simulink model "bms_master"  (R2024b)
settings: Solver=FixedStepDiscrete  StartTime=0.0  StopTime=T_stop  FixedStep=0.1  RelTol=1e-3
undefined symbols (not defined in the file): bms, C1_data, C2_data, dt, ekf_params, OCV_data, P_chiller_max, P_heater_max, Q_nom_Ah, R0_data, R1_data, R2_data, SoC_bp_ecm, SoC_bp_ocv, T_bp, T_cool_off, T_cool_on, T_cool_target, T_heat_off, T_heat_on, T_heat_target
libraries: simulink x28, components x12
settings Model: DataDictionary=buses.sldd  Creator=rayen  LastModifiedBy=rayen
settings OptimizationCC: DefaultParameterBehavior=Inlined  EnhancedBackFolding=on  PassReuseOutputArgsAs=Individual arguments  ZeroExternalMemoryAtStartup=off  ZeroInternalMemoryAtStartup=off  OptimizeBlockOrder=speed  DifferentSizesBufferReuse=on  OptimizationCustomize=off  EfficientTunableParamExpr=on
settings DebuggingCC: AlgebraicLoopMsg=error  ParameterTunabilityLossMsg=error
settings HardwareCC: TargetBitPerPointer=64  TargetBitPerSizeT=64  TargetBitPerPtrDiffT=64  TargetLargestAtomicFloat=Float  TargetIntDivRoundTo=Zero  TargetEndianess=LittleEndian  TargetWordSize=64  TargetHWDeviceType=Intel->x86-64 (Windows64)  ProdEqTarget=off
settings SFSimCC: MATLABDynamicMemAlloc=off  SimTargetLang=C++
settings RTWCC: Description=Embedded Coder  SystemTargetFile=ert.tlc  TemplateMakefile=ert_default_tmf
settings CodeAppCC: ForceParamTrailComments=on  IgnoreCustomStorageClasses=off  OperatorAnnotations=on  SimulinkDataObjDesc=on  SFDataObjDesc=on  InsertBlockDesc=on
settings ERTTargetCC: TargetLangStandard=C99 (ISO)  GenerateSampleERTMain=on  ERTCustomFileTemplate=example_file_process.tlc

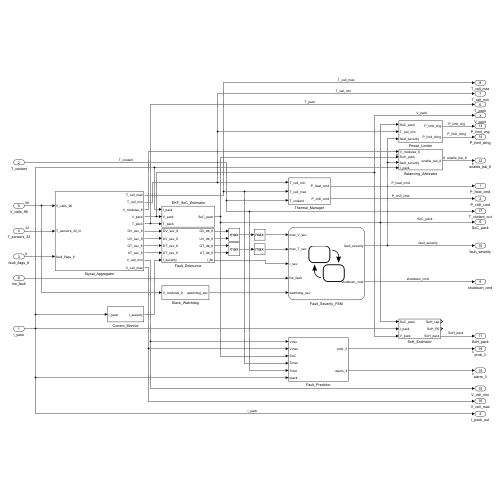
[thumbnail: Simulink's stored preview of the top-level diagram]
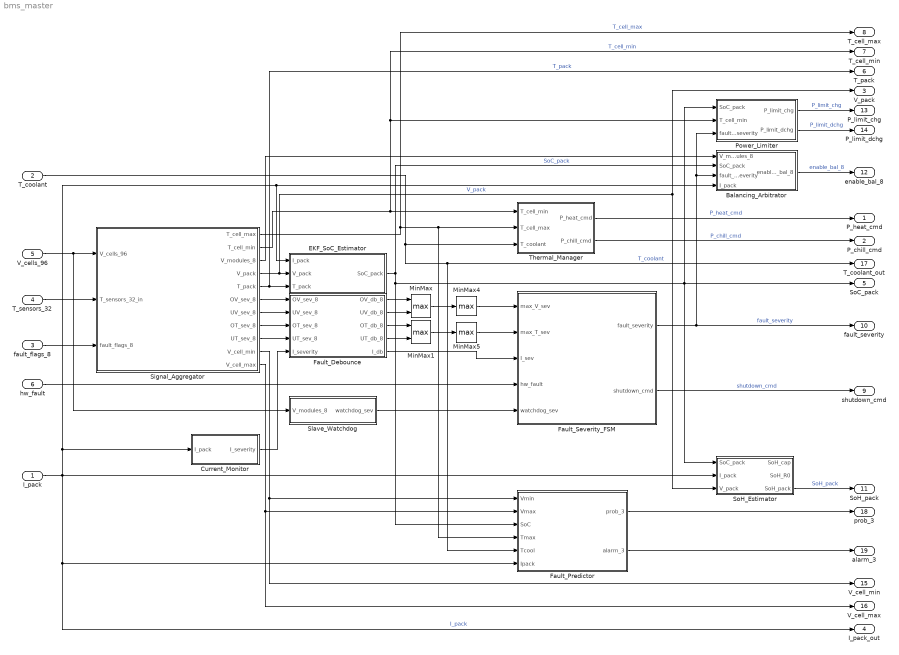
== system bms_master ==
  I_pack : Inport  OutDataTypeStr=double  PortDimensions=1
  T_coolant : Inport  Port=2  OutDataTypeStr=double  PortDimensions=1
  fault_flags_8 : Inport  Port=3  OutDataTypeStr=double  PortDimensions=[8]
  T_sensors_32 : Inport  Port=4  OutDataTypeStr=double  PortDimensions=[32]
  V_cells_96 : Inport  Port=5  OutDataTypeStr=double  PortDimensions=[96]
  hw_fault : Inport  Port=6
  " EKF_SoC_Estimator" : Subsystem
  Balancing_Arbitrator : Subsystem
  Current_Monitor : Subsystem
  Fault_Debounce : Subsystem
  Fault_Predictor : Subsystem
  Fault_Severity_FSM : Stateflow chart  TreatAsAtomicUnit=on
  MinMax : MinMax  Function=max  Inputs=2
  MinMax1 : MinMax  Function=max  Inputs=2
  MinMax4 : MinMax  Function=max
  MinMax5 : MinMax  Function=max
  Power_Limiter : Subsystem
  Signal_Aggregator : Subsystem
  Slave_Watchdog : Subsystem
  SoH_Estimator : Subsystem
  Thermal_Manager : Subsystem
  P_heat_cmd : Outport  OutDataTypeStr=double  PortDimensions=1
  P_chill_cmd : Outport  Port=2  OutDataTypeStr=double  PortDimensions=1
  V_pack : Outport  Port=3  OutDataTypeStr=double  PortDimensions=1
  I_pack_out : Outport  Port=4  OutDataTypeStr=double  PortDimensions=1
  SoC_pack : Outport  Port=5  OutDataTypeStr=double  PortDimensions=1
  T_pack : Outport  Port=6  OutDataTypeStr=double  PortDimensions=1
  T_cell_min : Outport  Port=7  OutDataTypeStr=double  PortDimensions=1
  T_cell_max : Outport  Port=8  OutDataTypeStr=double  PortDimensions=1
  shutdown_cmd : Outport  Port=9  OutDataTypeStr=double  PortDimensions=1
  fault_severity : Outport  Port=10  OutDataTypeStr=double  PortDimensions=1
  SoH_pack : Outport  Port=11  OutDataTypeStr=double  PortDimensions=1
  enable_bal_8 : Outport  Port=12  OutDataTypeStr=double  PortDimensions=[8]
  P_limit_chg : Outport  Port=13  OutDataTypeStr=double  PortDimensions=1
  P_limit_dchg : Outport  Port=14  OutDataTypeStr=double  PortDimensions=1
  V_cell_min : Outport  Port=15
  V_cell_max : Outport  Port=16
  T_coolant_out : Outport  Port=17
  prob_3 : Outport  Port=18  PortDimensions=[3]
  alarm_3 : Outport  Port=19  PortDimensions=[3]
  wires:
  Signal_Aggregator/6(OV_sev_8) -> Fault_Debounce/1(OV_sev_8)
  Signal_Aggregator/7(UV_sev_8) -> Fault_Debounce/2(UV_sev_8)
  Signal_Aggregator/8(OT_sev_8) -> Fault_Debounce/3(OT_sev_8)
  Signal_Aggregator/9(UT_sev_8) -> Fault_Debounce/4(UT_sev_8)
  Fault_Debounce/1(OV_db_8) -> MinMax/1
  Fault_Debounce/2(UV_db_8) -> MinMax/2
  Fault_Debounce/3(OT_db_8) -> MinMax1/1
  Fault_Debounce/4(UT_db_8) -> MinMax1/2
  MinMax/1 -> MinMax4/1
  MinMax1/1 -> MinMax5/1
  MinMax4/1 -> Fault_Severity_FSM/1(max_V_sev)
  MinMax5/1 -> Fault_Severity_FSM/2(max_T_sev)
  Slave_Watchdog/1(watchdog_sev) -> Fault_Severity_FSM/5(watchdog_sev)
  Signal_Aggregator/2(T_cell_min) -> Thermal_Manager/1(T_cell_min), T_cell_min/1, Power_Limiter/2(T_cell_min)  "T_cell_min"
  Signal_Aggregator/1(T_cell_max) -> T_cell_max/1, Thermal_Manager/2(T_cell_max), Fault_Predictor/4(Tmax)  "T_cell_max"
  Thermal_Manager/1(P_heat_cmd) -> P_heat_cmd/1  "P_heat_cmd"
  Thermal_Manager/2(P_chill_cmd) -> P_chill_cmd/1  "P_chill_cmd"
  T_coolant/1 -> Fault_Predictor/5(Tcool), T_coolant_out/1, Thermal_Manager/3(T_coolant)  "T_coolant"
  Signal_Aggregator/3(V_modules_8) -> Balancing_Arbitrator/1(V_modules_8)
  Fault_Severity_FSM/1(fault_severity) -> fault_severity/1, Power_Limiter/3(fault_severity), Balancing_Arbitrator/3(fault_severity)  "fault_severity"
  I_pack/1 -> I_pack_out/1, Fault_Predictor/6(Ipack), Current_Monitor/1(I_pack), Balancing_Arbitrator/4(I_pack), " EKF_SoC_Estimator"/1(I_pack), SoH_Estimator/2(I_pack)  "I_pack"
  Balancing_Arbitrator/1(enable_bal_8) -> enable_bal_8/1  "enable_bal_8"
  " EKF_SoC_Estimator"/1(SoC_pack) -> Fault_Predictor/3(SoC), Power_Limiter/1(SoC_pack), SoH_Estimator/1(SoC_pack), SoC_pack/1, Balancing_Arbitrator/2(SoC_pack)  "SoC_pack"
  Power_Limiter/1(P_limit_chg) -> P_limit_chg/1  "P_limit_chg"
  Power_Limiter/2(P_limit_dchg) -> P_limit_dchg/1  "P_limit_dchg"
  Fault_Severity_FSM/2(shutdown_cmd) -> shutdown_cmd/1  "shutdown_cmd"
  Signal_Aggregator/4(V_pack) -> " EKF_SoC_Estimator"/2(V_pack), SoH_Estimator/3(V_pack), V_pack/1  "V_pack"
  SoH_Estimator/3(SoH_pack) -> SoH_pack/1  "SoH_pack"
  Signal_Aggregator/5(T_pack) -> T_pack/1, " EKF_SoC_Estimator"/3(T_pack)  "T_pack"
  V_cells_96/1 -> Slave_Watchdog/1(V_modules_8), Signal_Aggregator/1(V_cells_96)
  Fault_Debounce/5(I_db) -> Fault_Severity_FSM/3(I_sev)
  T_sensors_32/1 -> Signal_Aggregator/2(T_sensors_32_in)
  fault_flags_8/1 -> Signal_Aggregator/3(fault_flags_8)
  hw_fault/1 -> Fault_Severity_FSM/4(hw_fault)
  Signal_Aggregator/11(V_cell_max) -> Fault_Predictor/2(Vmax), V_cell_max/1
  Signal_Aggregator/10(V_cell_min) -> Fault_Predictor/1(Vmin), V_cell_min/1
  Current_Monitor/1(I_severity) -> Fault_Debounce/5(I_severity)
  Fault_Predictor/1(prob_3) -> prob_3/1
  Fault_Predictor/2(alarm_3) -> alarm_3/1

== system bms_master/ EKF_SoC_Estimator ==
  I_pack : Inport
  V_pack : Inport  Port=2
  T_pack : Inport  Port=3
  Constant : Constant  Value=96
  MATLAB Function : MATLAB Function  TreatAsAtomicUnit=on
  SoC_pack : Outport
  wires:
  V_pack/1 -> MATLAB Function/1(V_pack)
  I_pack/1 -> MATLAB Function/2(I_pack)
  T_pack/1 -> MATLAB Function/3(T_pack)
  MATLAB Function/1(SoC_pack) -> SoC_pack/1
  Constant/1 -> MATLAB Function/4(N_series)

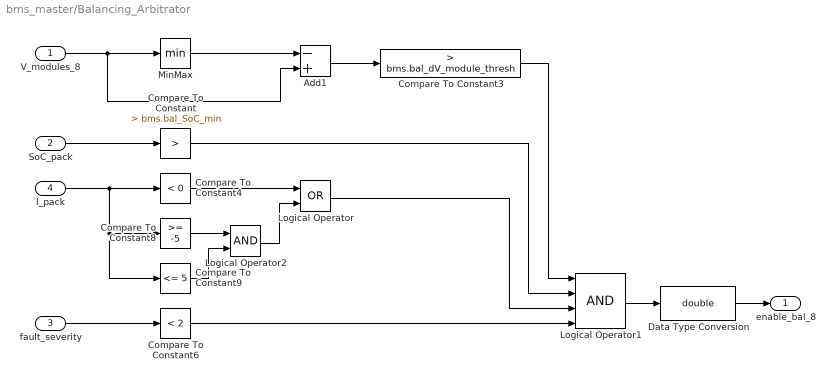
== system bms_master/Balancing_Arbitrator ==
  V_modules_8 : Inport  PortDimensions=[8]
  SoC_pack : Inport  Port=2
  fault_severity : Inport  Port=3  PortDimensions=[1]
  I_pack : Inport  Port=4
  Add1 : Sum  Inputs=-+
  Compare To Constant : simulink/Logic and Bit Operations/Compare To Constant  relop=>  const=bms.bal_SoC_min  OutDataTypeStr=boolean
  Compare To Constant3 : simulink/Logic and Bit Operations/Compare To Constant  relop=>  const=bms.bal_dV_module_thresh  OutDataTypeStr=boolean
  Compare To Constant4 : simulink/Logic and Bit Operations/Compare To Constant  relop=<  const=0  OutDataTypeStr=boolean
  Compare To Constant6 : simulink/Logic and Bit Operations/Compare To Constant  relop=<  const=2  OutDataTypeStr=boolean
  Compare To Constant8 : simulink/Logic and Bit Operations/Compare To Constant  relop=>=  const=-5  OutDataTypeStr=boolean
  Compare To Constant9 : simulink/Logic and Bit Operations/Compare To Constant  relop=<=  const=5  OutDataTypeStr=boolean
  Data Type Conversion : DataTypeConversion  OutDataTypeStr=double  SaturateOnIntegerOverflow=off  RndMeth=Floor
  Logical Operator : Logic  Operator=OR  AllPortsSameDT=off  OutDataTypeStr=boolean
  Logical Operator1 : Logic  Inputs=4  AllPortsSameDT=off  OutDataTypeStr=boolean
  Logical Operator2 : Logic  AllPortsSameDT=off  OutDataTypeStr=boolean
  MinMax : MinMax
  enable_bal_8 : Outport  PortDimensions=[8]
  wires:
  SoC_pack/1 -> Compare To Constant/1
  V_modules_8/1 -> MinMax/1, Add1/2
  I_pack/1 -> Compare To Constant9/1, Compare To Constant8/1, Compare To Constant4/1
  fault_severity/1 -> Compare To Constant6/1
  Compare To Constant8/1 -> Logical Operator2/1
  Compare To Constant9/1 -> Logical Operator2/2
  Compare To Constant4/1 -> Logical Operator/1
  Logical Operator2/1 -> Logical Operator/2
  Logical Operator1/1 -> Data Type Conversion/1
  Data Type Conversion/1 -> enable_bal_8/1
  MinMax/1 -> Add1/1
  Add1/1 -> Compare To Constant3/1
  Compare To Constant6/1 -> Logical Operator1/4
  Compare To Constant3/1 -> Logical Operator1/1
  Compare To Constant/1 -> Logical Operator1/2
  Logical Operator/1 -> Logical Operator1/3

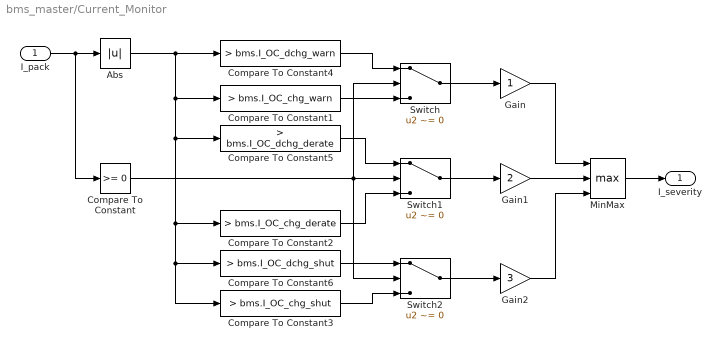
== system bms_master/Current_Monitor ==
  I_pack : Inport
  Abs : Abs  SaturateOnIntegerOverflow=off
  Compare To Constant : simulink/Logic and Bit Operations/Compare To Constant  relop=>=  const=0  OutDataTypeStr=boolean
  Compare To Constant1 : simulink/Logic and Bit Operations/Compare To Constant  relop=>  const=bms.I_OC_chg_warn  OutDataTypeStr=boolean
  Compare To Constant2 : simulink/Logic and Bit Operations/Compare To Constant  relop=>  const=bms.I_OC_chg_derate  OutDataTypeStr=boolean
  Compare To Constant3 : simulink/Logic and Bit Operations/Compare To Constant  relop=>  const=bms.I_OC_chg_shut  OutDataTypeStr=boolean
  Compare To Constant4 : simulink/Logic and Bit Operations/Compare To Constant  relop=>  const=bms.I_OC_dchg_warn  OutDataTypeStr=boolean
  Compare To Constant5 : simulink/Logic and Bit Operations/Compare To Constant  relop=>  const=bms.I_OC_dchg_derate  OutDataTypeStr=boolean
  Compare To Constant6 : simulink/Logic and Bit Operations/Compare To Constant  relop=>  const=bms.I_OC_dchg_shut  OutDataTypeStr=boolean
  Gain : Gain
  Gain1 : Gain  Gain=2
  Gain2 : Gain  Gain=3
  MinMax : MinMax  Function=max  Inputs=3
  Switch : Switch  Criteria=u2 ~= 0  SaturateOnIntegerOverflow=off  InputSameDT=off
  Switch1 : Switch  Criteria=u2 ~= 0  SaturateOnIntegerOverflow=off  InputSameDT=off
  Switch2 : Switch  Criteria=u2 ~= 0  SaturateOnIntegerOverflow=off  InputSameDT=off
  I_severity : Outport
  wires:
  Switch/1 -> Gain/1
  I_pack/1 -> Compare To Constant/1, Abs/1
  Abs/1 -> Compare To Constant6/1, Compare To Constant3/1, Compare To Constant2/1, Compare To Constant5/1, Compare To Constant1/1, Compare To Constant4/1
  Compare To Constant4/1 -> Switch/1
  Compare To Constant5/1 -> Switch1/1
  Compare To Constant6/1 -> Switch2/1
  Gain/1 -> MinMax/1
  Switch2/1 -> Gain2/1
  Compare To Constant1/1 -> Switch/3
  Compare To Constant3/1 -> Switch2/3
  Compare To Constant2/1 -> Switch1/3
  Switch1/1 -> Gain1/1
  Gain1/1 -> MinMax/2
  Gain2/1 -> MinMax/3
  MinMax/1 -> I_severity/1
  Compare To Constant/1 -> Switch1/2, Switch2/2, Switch/2

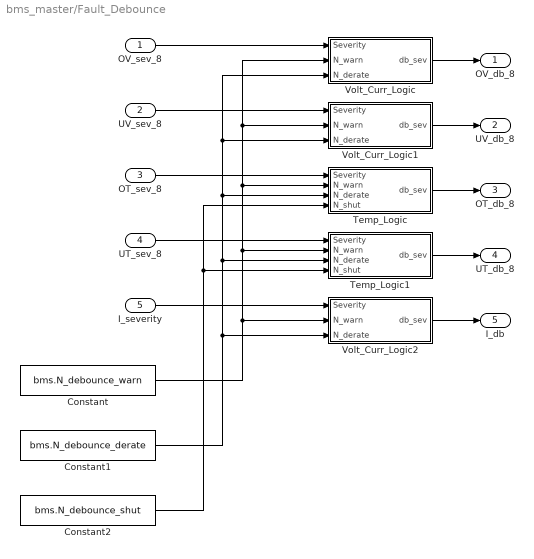
== system bms_master/Fault_Debounce ==
  OV_sev_8 : Inport
  UV_sev_8 : Inport  Port=2
  OT_sev_8 : Inport  Port=3
  UT_sev_8 : Inport  Port=4
  I_severity : Inport  Port=5
  Constant : Constant  Value=bms.N_debounce_warn
  Constant1 : Constant  Value=bms.N_debounce_derate
  Constant2 : Constant  Value=bms.N_debounce_shut
  Temp_Logic : Subsystem
  Temp_Logic1 : Subsystem
  Volt_Curr_Logic : Subsystem
  Volt_Curr_Logic1 : Subsystem
  Volt_Curr_Logic2 : Subsystem
  OV_db_8 : Outport
  UV_db_8 : Outport  Port=2
  OT_db_8 : Outport  Port=3
  UT_db_8 : Outport  Port=4
  I_db : Outport  Port=5
  wires:
  OV_sev_8/1 -> Volt_Curr_Logic/1(Severity)
  Constant/1 -> Temp_Logic1/2(N_warn), Temp_Logic/2(N_warn), Volt_Curr_Logic/2(N_warn), Volt_Curr_Logic1/2(N_warn), Volt_Curr_Logic2/2(N_warn)
  Constant1/1 -> Volt_Curr_Logic/3(N_derate), Volt_Curr_Logic1/3(N_derate), Temp_Logic/3(N_derate), Temp_Logic1/3(N_derate), Volt_Curr_Logic2/3(N_derate)
  UV_sev_8/1 -> Volt_Curr_Logic1/1(Severity)
  I_severity/1 -> Volt_Curr_Logic2/1(Severity)
  OT_sev_8/1 -> Temp_Logic/1(Severity)
  Constant2/1 -> Temp_Logic1/4(N_shut), Temp_Logic/4(N_shut)
  UT_sev_8/1 -> Temp_Logic1/1(Severity)
  Volt_Curr_Logic/1(db_sev) -> OV_db_8/1
  Volt_Curr_Logic1/1(db_sev) -> UV_db_8/1
  Temp_Logic/1(db_sev) -> OT_db_8/1
  Temp_Logic1/1(db_sev) -> UT_db_8/1
  Volt_Curr_Logic2/1(db_sev) -> I_db/1

== system bms_master/Fault_Predictor ==
  Vmin : Inport
  Vmax : Inport  Port=2
  SoC : Inport  Port=3
  Tmax : Inport  Port=4
  Tcool : Inport  Port=5
  Ipack : Inport  Port=6
  fault_predictor : ModelReference  ModelNameDialog=fault_predictor.slx  SimulationMode=Normal  ModelReferenceVersion=1.72
  prob_3 : Outport
  alarm_3 : Outport  Port=2
  wires:
  Vmin/1 -> fault_predictor/1
  Tcool/1 -> fault_predictor/5
  SoC/1 -> fault_predictor/3
  Vmax/1 -> fault_predictor/2
  Tmax/1 -> fault_predictor/4
  Ipack/1 -> fault_predictor/6
  fault_predictor/1 -> prob_3/1
  fault_predictor/2 -> alarm_3/1

== system bms_master/Power_Limiter ==
  SoC_pack : Inport
  T_cell_min : Inport  Port=2
  fault_severity : Inport  Port=3
  P_base : Subsystem
  Product : Product  Inputs=3
  Product3 : Product  Inputs=3
  k_severity : Lookup_n-D  NumberOfTableDimensions=1  BreakpointsForDimension1=[0, 1, 2, 3]  Table=[1.0, 1.0, 0.5, 0]  InternalRulePriority=Speed  RndMeth=Simplest
  min(k_soc,k_temp) : Subsystem
  P_limit_chg : Outport
  P_limit_dchg : Outport  Port=2
  wires:
  SoC_pack/1 -> min(k_soc,k_temp)/1(SoC_pack)
  T_cell_min/1 -> min(k_soc,k_temp)/2(T_cell_min)
  fault_severity/1 -> k_severity/1
  k_severity/1 -> Product3/3, Product/3
  P_base/2(P_base_dchg) -> Product3/2
  min(k_soc,k_temp)/2(min_dchg) -> Product3/1
  P_base/1(P_base_chg) -> Product/2
  min(k_soc,k_temp)/1(min_chg) -> Product/1
  Product3/1 -> P_limit_dchg/1
  Product/1 -> P_limit_chg/1

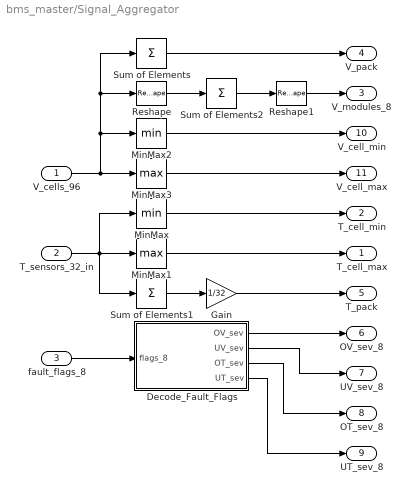
== system bms_master/Signal_Aggregator ==
  V_cells_96 : Inport
  T_sensors_32_in : Inport  Port=2
  fault_flags_8 : Inport  Port=3
  Decode_Fault_Flags : Subsystem
  Gain : Gain  Gain=1/32
  MinMax : MinMax
  MinMax1 : MinMax  Function=max
  MinMax2 : MinMax
  MinMax3 : MinMax  Function=max
  Reshape : Reshape  OutputDimensionality=Customize  OutputDimensions=[12, 8]
  Reshape1 : Reshape  OutputDimensionality=Customize  OutputDimensions=[8, 1]
  Sum of Elements : Sum  Inputs=+
  Sum of Elements1 : Sum  Inputs=+
  Sum of Elements2 : Sum  Inputs=+  CollapseMode=Specified dimension
  T_cell_max : Outport
  T_cell_min : Outport  Port=2
  V_modules_8 : Outport  Port=3
  V_pack : Outport  Port=4
  T_pack : Outport  Port=5
  OV_sev_8 : Outport  Port=6
  UV_sev_8 : Outport  Port=7
  OT_sev_8 : Outport  Port=8
  UT_sev_8 : Outport  Port=9
  V_cell_min : Outport  Port=10
  V_cell_max : Outport  Port=11
  wires:
  V_cells_96/1 -> MinMax3/1, MinMax2/1, Reshape/1, Sum of Elements/1
  Sum of Elements/1 -> V_pack/1
  T_sensors_32_in/1 -> MinMax1/1, MinMax/1, Sum of Elements1/1
  MinMax/1 -> T_cell_min/1
  MinMax1/1 -> T_cell_max/1
  Sum of Elements1/1 -> Gain/1
  Gain/1 -> T_pack/1
  fault_flags_8/1 -> Decode_Fault_Flags/1(flags_8)
  Decode_Fault_Flags/1(OV_sev) -> OV_sev_8/1
  Decode_Fault_Flags/2(UV_sev) -> UV_sev_8/1
  Decode_Fault_Flags/3(OT_sev) -> OT_sev_8/1
  Decode_Fault_Flags/4(UT_sev) -> UT_sev_8/1
  MinMax2/1 -> V_cell_min/1
  MinMax3/1 -> V_cell_max/1
  Reshape1/1 -> V_modules_8/1
  Reshape/1 -> Sum of Elements2/1
  Sum of Elements2/1 -> Reshape1/1

== system bms_master/Slave_Watchdog ==
  V_modules_8 : Inport
  Watchdog_Logic : Subsystem
  Watchdog_Severity : Subsystem
  watchdog_sev : Outport
  wires:
  Watchdog_Logic/1(status) -> Watchdog_Severity/1(status)
  V_modules_8/1 -> Watchdog_Logic/1(V_modules_8)
  Watchdog_Severity/1(watchdog_sev) -> watchdog_sev/1

== system bms_master/SoH_Estimator ==
  SoC_pack : Inport
  I_pack : Inport  Port=2
  V_pack : Inport  Port=3
  MATLAB Function : MATLAB Function  TreatAsAtomicUnit=on
  SoH_cap : Outport
  SoH_R0 : Outport  Port=2
  SoH_pack : Outport  Port=3
  wires:
  SoC_pack/1 -> MATLAB Function/1(SoC_pack)
  I_pack/1 -> MATLAB Function/2(I_pack)
  V_pack/1 -> MATLAB Function/3(V_pack)
  MATLAB Function/3(SoH_pack) -> SoH_pack/1
  MATLAB Function/2(SoH_R0) -> SoH_R0/1
  MATLAB Function/1(SoH_cap) -> SoH_cap/1

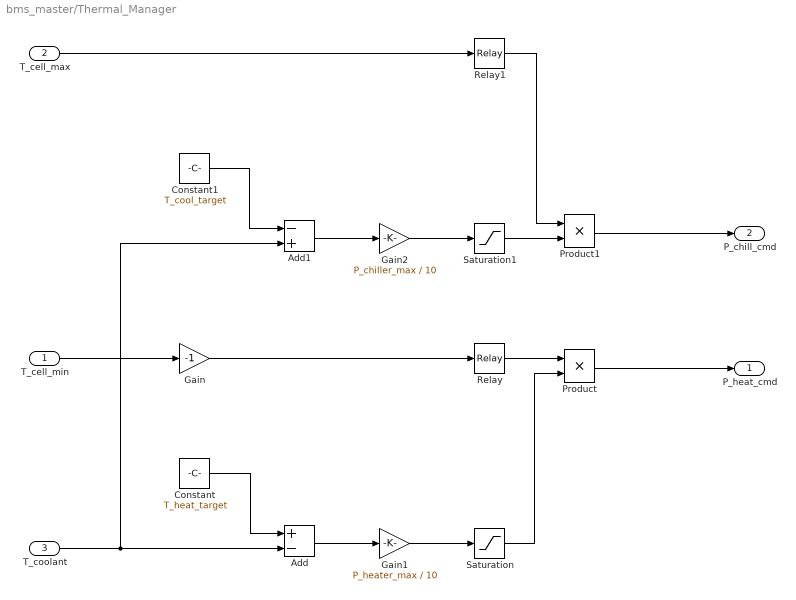
== system bms_master/Thermal_Manager ==
  T_cell_min : Inport
  T_cell_max : Inport  Port=2
  T_coolant : Inport  Port=3
  Add : Sum  Inputs=+-
  Add1 : Sum  Inputs=-+
  Constant : Constant  Value=T_heat_target
  Constant1 : Constant  Value=T_cool_target
  Gain : Gain  Gain=-1
  Gain1 : Gain  Gain=P_heater_max / 10
  Gain2 : Gain  Gain=P_chiller_max / 10
  Product : Product
  Product1 : Product
  Relay : Relay  OnSwitchValue=-T_heat_on  OffSwitchValue=-T_heat_off
  Relay1 : Relay  OnSwitchValue=T_cool_on  OffSwitchValue=T_cool_off
  Saturation : Saturate  UpperLimit=P_heater_max  LowerLimit=0
  Saturation1 : Saturate  UpperLimit=P_chiller_max  LowerLimit=0
  P_heat_cmd : Outport
  P_chill_cmd : Outport  Port=2
  wires:
  Product/1 -> P_heat_cmd/1
  Add1/1 -> Gain2/1
  Add/1 -> Gain1/1
  Gain/1 -> Relay/1
  Saturation1/1 -> Product1/2
  Constant/1 -> Add/1
  Constant1/1 -> Add1/1
  Gain2/1 -> Saturation1/1
  Relay1/1 -> Product1/1
  T_cell_min/1 -> Gain/1
  T_coolant/1 -> Add1/2, Add/2
  T_cell_max/1 -> Relay1/1
  Gain1/1 -> Saturation/1
  Product1/1 -> P_chill_cmd/1
  Saturation/1 -> Product/2
  Relay/1 -> Product/1

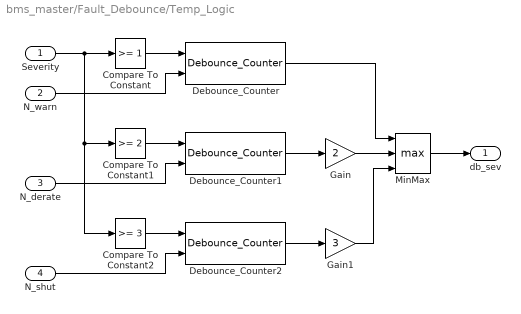
== system bms_master/Fault_Debounce/Temp_Logic ==
  Severity : Inport
  N_warn : Inport  Port=2
  N_derate : Inport  Port=3
  N_shut : Inport  Port=4
  Compare To Constant : simulink/Logic and Bit Operations/Compare To Constant  relop=>=  const=1  OutDataTypeStr=boolean
  Compare To Constant1 : simulink/Logic and Bit Operations/Compare To Constant  relop=>=  const=2  OutDataTypeStr=boolean
  Compare To Constant2 : simulink/Logic and Bit Operations/Compare To Constant  relop=>=  const=3  OutDataTypeStr=boolean
  Debounce_Counter : components/Debounce_Counter  SystemSampleTime=-1  VariantActivationTime=update diagram  AllowFlexibleInterface=on  Latency=0  AutoFrameSizeCalculation=off
  Debounce_Counter1 : components/Debounce_Counter  SystemSampleTime=-1  VariantActivationTime=update diagram  AllowFlexibleInterface=on  Latency=0  AutoFrameSizeCalculation=off
  Debounce_Counter2 : components/Debounce_Counter  SystemSampleTime=-1  VariantActivationTime=update diagram  AllowFlexibleInterface=on  Latency=0  AutoFrameSizeCalculation=off
  Gain : Gain  Gain=2
  Gain1 : Gain  Gain=3
  MinMax : MinMax  Function=max  Inputs=3
  db_sev : Outport
  wires:
  Compare To Constant/1 -> Debounce_Counter/1
  Compare To Constant2/1 -> Debounce_Counter2/1
  Compare To Constant1/1 -> Debounce_Counter1/1
  Severity/1 -> Compare To Constant/1, Compare To Constant2/1, Compare To Constant1/1
  N_warn/1 -> Debounce_Counter/2
  N_derate/1 -> Debounce_Counter1/2
  N_shut/1 -> Debounce_Counter2/2
  Debounce_Counter/1 -> MinMax/1
  Debounce_Counter1/1 -> Gain/1
  Debounce_Counter2/1 -> Gain1/1
  Gain/1 -> MinMax/2
  Gain1/1 -> MinMax/3
  MinMax/1 -> db_sev/1

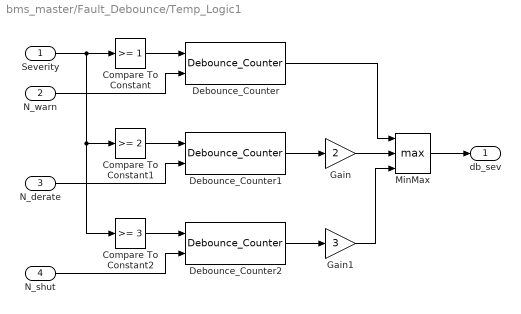
== system bms_master/Fault_Debounce/Temp_Logic1 ==
  Severity : Inport
  N_warn : Inport  Port=2
  N_derate : Inport  Port=3
  N_shut : Inport  Port=4
  Compare To Constant : simulink/Logic and Bit Operations/Compare To Constant  relop=>=  const=1  OutDataTypeStr=boolean
  Compare To Constant1 : simulink/Logic and Bit Operations/Compare To Constant  relop=>=  const=2  OutDataTypeStr=boolean
  Compare To Constant2 : simulink/Logic and Bit Operations/Compare To Constant  relop=>=  const=3  OutDataTypeStr=boolean
  Debounce_Counter : components/Debounce_Counter  SystemSampleTime=-1  VariantActivationTime=update diagram  AllowFlexibleInterface=on  Latency=0  AutoFrameSizeCalculation=off
  Debounce_Counter1 : components/Debounce_Counter  SystemSampleTime=-1  VariantActivationTime=update diagram  AllowFlexibleInterface=on  Latency=0  AutoFrameSizeCalculation=off
  Debounce_Counter2 : components/Debounce_Counter  SystemSampleTime=-1  VariantActivationTime=update diagram  AllowFlexibleInterface=on  Latency=0  AutoFrameSizeCalculation=off
  Gain : Gain  Gain=2
  Gain1 : Gain  Gain=3
  MinMax : MinMax  Function=max  Inputs=3
  db_sev : Outport
  wires:
  Compare To Constant/1 -> Debounce_Counter/1
  Compare To Constant2/1 -> Debounce_Counter2/1
  Compare To Constant1/1 -> Debounce_Counter1/1
  Severity/1 -> Compare To Constant/1, Compare To Constant2/1, Compare To Constant1/1
  N_warn/1 -> Debounce_Counter/2
  N_derate/1 -> Debounce_Counter1/2
  N_shut/1 -> Debounce_Counter2/2
  Debounce_Counter/1 -> MinMax/1
  Debounce_Counter1/1 -> Gain/1
  Debounce_Counter2/1 -> Gain1/1
  Gain/1 -> MinMax/2
  Gain1/1 -> MinMax/3
  MinMax/1 -> db_sev/1

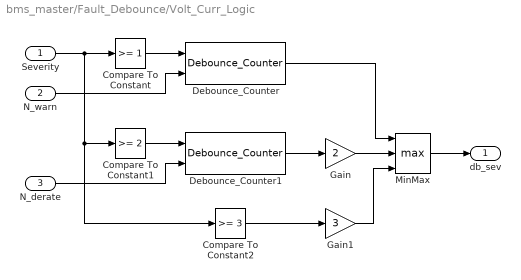
== system bms_master/Fault_Debounce/Volt_Curr_Logic ==
  Severity : Inport
  N_warn : Inport  Port=2
  N_derate : Inport  Port=3
  Compare To Constant : simulink/Logic and Bit Operations/Compare To Constant  relop=>=  const=1  OutDataTypeStr=boolean
  Compare To Constant1 : simulink/Logic and Bit Operations/Compare To Constant  relop=>=  const=2  OutDataTypeStr=boolean
  Compare To Constant2 : simulink/Logic and Bit Operations/Compare To Constant  relop=>=  const=3  OutDataTypeStr=boolean
  Debounce_Counter : components/Debounce_Counter  SystemSampleTime=-1  VariantActivationTime=update diagram  AllowFlexibleInterface=on  Latency=0  AutoFrameSizeCalculation=off
  Debounce_Counter1 : components/Debounce_Counter  SystemSampleTime=-1  VariantActivationTime=update diagram  AllowFlexibleInterface=on  Latency=0  AutoFrameSizeCalculation=off
  Gain : Gain  Gain=2
  Gain1 : Gain  Gain=3
  MinMax : MinMax  Function=max  Inputs=3
  db_sev : Outport
  wires:
  Debounce_Counter1/1 -> Gain/1
  Debounce_Counter/1 -> MinMax/1
  Severity/1 -> Compare To Constant2/1, Compare To Constant1/1, Compare To Constant/1
  MinMax/1 -> db_sev/1
  Compare To Constant/1 -> Debounce_Counter/1
  N_warn/1 -> Debounce_Counter/2
  Compare To Constant1/1 -> Debounce_Counter1/1
  N_derate/1 -> Debounce_Counter1/2
  Compare To Constant2/1 -> Gain1/1
  Gain/1 -> MinMax/2
  Gain1/1 -> MinMax/3

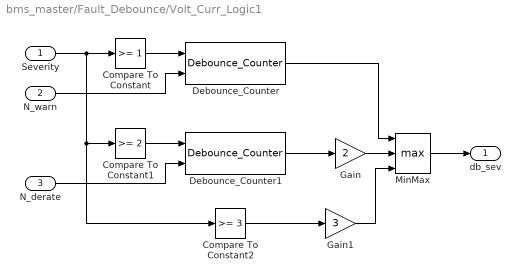
== system bms_master/Fault_Debounce/Volt_Curr_Logic1 ==
  Severity : Inport
  N_warn : Inport  Port=2
  N_derate : Inport  Port=3
  Compare To Constant : simulink/Logic and Bit Operations/Compare To Constant  relop=>=  const=1  OutDataTypeStr=boolean
  Compare To Constant1 : simulink/Logic and Bit Operations/Compare To Constant  relop=>=  const=2  OutDataTypeStr=boolean
  Compare To Constant2 : simulink/Logic and Bit Operations/Compare To Constant  relop=>=  const=3  OutDataTypeStr=boolean
  Debounce_Counter : components/Debounce_Counter  SystemSampleTime=-1  VariantActivationTime=update diagram  AllowFlexibleInterface=on  Latency=0  AutoFrameSizeCalculation=off
  Debounce_Counter1 : components/Debounce_Counter  SystemSampleTime=-1  VariantActivationTime=update diagram  AllowFlexibleInterface=on  Latency=0  AutoFrameSizeCalculation=off
  Gain : Gain  Gain=2
  Gain1 : Gain  Gain=3
  MinMax : MinMax  Function=max  Inputs=3
  db_sev : Outport
  wires:
  Debounce_Counter1/1 -> Gain/1
  Debounce_Counter/1 -> MinMax/1
  Severity/1 -> Compare To Constant2/1, Compare To Constant1/1, Compare To Constant/1
  MinMax/1 -> db_sev/1
  Compare To Constant/1 -> Debounce_Counter/1
  N_warn/1 -> Debounce_Counter/2
  Compare To Constant1/1 -> Debounce_Counter1/1
  N_derate/1 -> Debounce_Counter1/2
  Compare To Constant2/1 -> Gain1/1
  Gain/1 -> MinMax/2
  Gain1/1 -> MinMax/3

== system bms_master/Fault_Debounce/Volt_Curr_Logic2 ==
  Severity : Inport
  N_warn : Inport  Port=2
  N_derate : Inport  Port=3
  Compare To Constant : simulink/Logic and Bit Operations/Compare To Constant  relop=>=  const=1  OutDataTypeStr=boolean
  Compare To Constant1 : simulink/Logic and Bit Operations/Compare To Constant  relop=>=  const=2  OutDataTypeStr=boolean
  Compare To Constant2 : simulink/Logic and Bit Operations/Compare To Constant  relop=>=  const=3  OutDataTypeStr=boolean
  Debounce_Counter : components/Debounce_Counter  SystemSampleTime=-1  VariantActivationTime=update diagram  AllowFlexibleInterface=on  Latency=0  AutoFrameSizeCalculation=off
  Debounce_Counter1 : components/Debounce_Counter  SystemSampleTime=-1  VariantActivationTime=update diagram  AllowFlexibleInterface=on  Latency=0  AutoFrameSizeCalculation=off
  Gain : Gain  Gain=2
  Gain1 : Gain  Gain=3
  MinMax : MinMax  Function=max  Inputs=3
  db_sev : Outport
  wires:
  Debounce_Counter1/1 -> Gain/1
  Debounce_Counter/1 -> MinMax/1
  Severity/1 -> Compare To Constant2/1, Compare To Constant1/1, Compare To Constant/1
  MinMax/1 -> db_sev/1
  Compare To Constant/1 -> Debounce_Counter/1
  N_warn/1 -> Debounce_Counter/2
  Compare To Constant1/1 -> Debounce_Counter1/1
  N_derate/1 -> Debounce_Counter1/2
  Compare To Constant2/1 -> Gain1/1
  Gain/1 -> MinMax/2
  Gain1/1 -> MinMax/3

== system bms_master/Power_Limiter/P_base ==
  Constant : Constant  Value=96
  I_chg_max : Constant  Value=150
  I_dchg_max : Constant  Value=405
  Product : Product  Inputs=3
  Product1 : Product  Inputs=3
  V_cell_max : Constant  Value=4.2
  V_cell_max_dchg : Constant  Value=4.2
  P_base_chg : Outport
  P_base_dchg : Outport  Port=2
  wires:
  I_chg_max/1 -> Product/1
  Constant/1 -> Product/3, Product1/1
  V_cell_max/1 -> Product/2
  I_dchg_max/1 -> Product1/2
  V_cell_max_dchg/1 -> Product1/3
  Product/1 -> P_base_chg/1
  Product1/1 -> P_base_dchg/1

== system bms_master/Power_Limiter/min(k_soc,k_temp) ==
  SoC_pack : Inport
  T_cell_min : Inport  Port=2
  MinMax2 : MinMax  Inputs=2
  MinMax3 : MinMax  Inputs=2
  SoC_chg_derating : Lookup_n-D  NumberOfTableDimensions=1  BreakpointsForDimension1=[0.85, 0.93, 0.97, 1.00]  Table=[1.0, 0.5, 0.2, 0]  InternalRulePriority=Speed  RndMeth=Simplest
  SoC_dchg_derating : Lookup_n-D  NumberOfTableDimensions=1  BreakpointsForDimension1=[0, 0.05, 0.10, 0.20]  Table=[0, 0.3, 0.7, 1.0]  InternalRulePriority=Speed  RndMeth=Simplest
  T_chg_derating : Lookup_n-D  NumberOfTableDimensions=1  BreakpointsForDimension1=[-20, -10, 0, 10, 25, 45, 55]  Table=[0, 0, 0.1, 0.4, 1.0, 1.0, 0]  InternalRulePriority=Speed  RndMeth=Simplest
  T_dchg_derating : Lookup_n-D  NumberOfTableDimensions=1  BreakpointsForDimension1=[-20, -10, 50, 60]  Table=[0, 1.0, 1.0, 0]  InternalRulePriority=Speed  RndMeth=Simplest
  min_chg : Outport
  min_dchg : Outport  Port=2
  wires:
  T_cell_min/1 -> T_chg_derating/1, T_dchg_derating/1
  MinMax3/1 -> min_dchg/1
  MinMax2/1 -> min_chg/1
  SoC_pack/1 -> SoC_chg_derating/1, SoC_dchg_derating/1
  T_chg_derating/1 -> MinMax2/1
  SoC_dchg_derating/1 -> MinMax3/2
  SoC_chg_derating/1 -> MinMax2/2
  T_dchg_derating/1 -> MinMax3/1

== system bms_master/Signal_Aggregator/Decode_Fault_Flags ==
  flags_8 : Inport
  decode_bits : MATLAB Function  TreatAsAtomicUnit=on
  OV_sev : Outport
  UV_sev : Outport  Port=2
  OT_sev : Outport  Port=3
  UT_sev : Outport  Port=4
  wires:
  flags_8/1 -> decode_bits/1(flags_8)
  decode_bits/1(OV_sev) -> OV_sev/1
  decode_bits/2(UV_sev) -> UV_sev/1
  decode_bits/3(OT_sev) -> OT_sev/1
  decode_bits/4(UT_sev) -> UT_sev/1

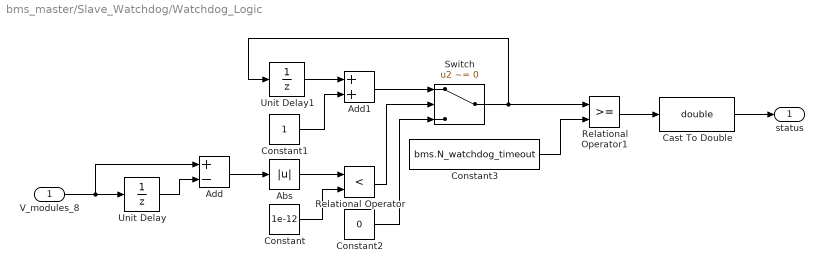
== system bms_master/Slave_Watchdog/Watchdog_Logic ==
  V_modules_8 : Inport
  Abs : Abs  SaturateOnIntegerOverflow=off
  Add : Sum  Inputs=+-
  Add1 : Sum
  Cast To Double : DataTypeConversion  OutDataTypeStr=double  SaturateOnIntegerOverflow=off  RndMeth=Floor
  Constant : Constant  Value=1e-12
  Constant1 : Constant
  Constant2 : Constant  Value=0
  Constant3 : Constant  Value=bms.N_watchdog_timeout
  Relational Operator : RelationalOperator  Operator=<  OutDataTypeStr=boolean  RndMeth=Simplest  InputSameDT=off
  Relational Operator1 : RelationalOperator  OutDataTypeStr=boolean  RndMeth=Simplest  InputSameDT=off
  Switch : Switch  Criteria=u2 ~= 0  SaturateOnIntegerOverflow=off  InputSameDT=off
  Unit Delay : UnitDelay  SampleTime=dt  HasFrameUpgradeWarning=on
  Unit Delay1 : UnitDelay  SampleTime=dt  HasFrameUpgradeWarning=on
  status : Outport
  wires:
  Unit Delay/1 -> Add/2
  V_modules_8/1 -> Add/1, Unit Delay/1
  Constant3/1 -> Relational Operator1/2
  Add1/1 -> Switch/1
  Constant1/1 -> Add1/2
  Add/1 -> Abs/1
  Relational Operator/1 -> Switch/2
  Constant/1 -> Relational Operator/2
  Unit Delay1/1 -> Add1/1
  Abs/1 -> Relational Operator/1
  Constant2/1 -> Switch/3
  Switch/1 -> Unit Delay1/1, Relational Operator1/1
  Relational Operator1/1 -> Cast To Double/1
  Cast To Double/1 -> status/1

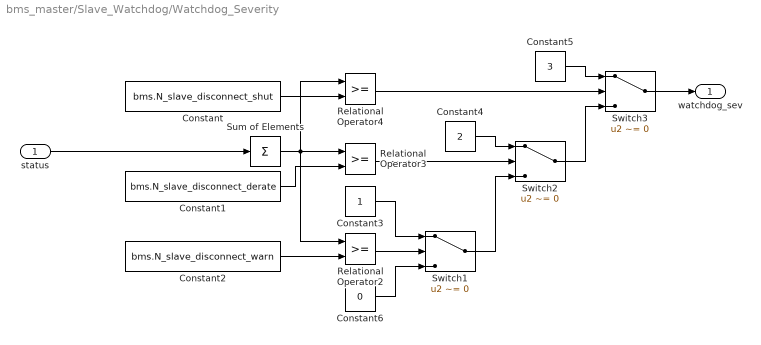
== system bms_master/Slave_Watchdog/Watchdog_Severity ==
  status : Inport
  Constant : Constant  Value=bms.N_slave_disconnect_shut
  Constant1 : Constant  Value=bms.N_slave_disconnect_derate
  Constant2 : Constant  Value=bms.N_slave_disconnect_warn
  Constant3 : Constant
  Constant4 : Constant  Value=2
  Constant5 : Constant  Value=3
  Constant6 : Constant  Value=0
  Relational Operator2 : RelationalOperator  OutDataTypeStr=boolean  RndMeth=Simplest  InputSameDT=off
  Relational Operator3 : RelationalOperator  OutDataTypeStr=boolean  RndMeth=Simplest  InputSameDT=off
  Relational Operator4 : RelationalOperator  OutDataTypeStr=boolean  RndMeth=Simplest  InputSameDT=off
  Sum of Elements : Sum  Inputs=+
  Switch1 : Switch  Criteria=u2 ~= 0  SaturateOnIntegerOverflow=off  InputSameDT=off
  Switch2 : Switch  Criteria=u2 ~= 0  SaturateOnIntegerOverflow=off  InputSameDT=off
  Switch3 : Switch  Criteria=u2 ~= 0  SaturateOnIntegerOverflow=off  InputSameDT=off
  watchdog_sev : Outport
  wires:
  Constant3/1 -> Switch1/1
  Switch3/1 -> watchdog_sev/1
  Constant2/1 -> Relational Operator2/2
  Constant4/1 -> Switch2/1
  status/1 -> Sum of Elements/1
  Constant/1 -> Relational Operator4/2
  Sum of Elements/1 -> Relational Operator3/1, Relational Operator4/1, Relational Operator2/1
  Constant1/1 -> Relational Operator3/2
  Relational Operator3/1 -> Switch2/2
  Relational Operator4/1 -> Switch3/2
  Relational Operator2/1 -> Switch1/2
  Constant6/1 -> Switch1/3
  Switch1/1 -> Switch2/3
  Switch2/1 -> Switch3/3
  Constant5/1 -> Switch3/1

== matlab function bms_master/SoH_Estimator/MATLAB Function ==
  data: SoC_pack input; SoH_cap output; I_pack input; V_pack input; SoH_R0 output; SoH_pack output; OCV_data parameter; Q_nom_Ah parameter; dt parameter; SoC_bp_ocv parameter; bms parameter
function [SoH_cap, SoH_R0, SoH_pack] = soh_estimator_fcn( ...
        SoC_pack, I_pack, V_pack, OCV_data, ...
        Q_nom_Ah, dt, SoC_bp_ocv, bms)
  %#codegen
  % --- Persistent state ---
  persistent SoC_start Q_acc SoH_cap_est R0_ema
  if isempty(SoC_start)
      SoC_start    = SoC_pack;
      Q_acc        = 0;
      SoH_cap_est  = bms.SoH_init;   % carry-over from previous trip
      R0_ema       = bms.R0_fresh;
  end

  % --- 1) Coulomb-counting capacity ---
  Q_acc = Q_acc + abs(I_pack) * dt / 3600;   % [Ah]
  dSoC  = abs(SoC_pack - SoC_start) * 100;   % [%%]

  if dSoC >= bms.dSoC_min_pct                     % deep enough swing
      Q_expected  = (dSoC / 100) * Q_nom_Ah;
      SoH_cap_est = min(1, Q_acc / Q_expected);
      % reset for next window
      SoC_start    = SoC_pack;
      Q_acc        = 0;
  end

  % --- 2) R0 trend (EMA) ---
  if abs(I_pack) > 5   % avoid division by near-zero current
      % Use OCV at 25 degC (column 6 of OCV_data)
      V_oc_est = interp1_lut(SoC_bp_ocv, OCV_data(:,6), SoC_pack * 100);
      R0_inst  = abs((V_pack / 96) - V_oc_est) / abs(I_pack);
      R0_ema   = bms.alpha_ema * R0_inst + (1 - bms.alpha_ema) * R0_ema;
  end
  SoH_R0 = min(1, max(0, 2 - R0_ema / bms.R0_fresh));  % linear map

  % --- 3) Combined SoH ---
  SoH_cap = SoH_cap_est;
  SoH_pack = SoH_cap;   % capacity-based; SoH_R0 available separately

end
function v = interp1_lut(xbp, ydata, xq)
%INTERP1_LUT  Codegen-safe 1-D linear interpolation.
  xq = max(xbp(1), min(xbp(end), xq));
  ix = int32(1);
  for k = 1:int32(numel(xbp)-1)
      if xq >= xbp(k), ix = k; end
  end
  ix2 = min(ix+1, int32(numel(xbp)));
  if ix == ix2
      v = ydata(ix);
  else
      fx = (xq - xbp(ix)) / (xbp(ix2) - xbp(ix));
      v = ydata(ix) * (1 - fx) + ydata(ix2) * fx;
  end
end

== matlab function bms_master/ EKF_SoC_Estimator/MATLAB Function ==
  data: V_pack input; I_pack input; T_pack input; OCV_data parameter; R0_data parameter; R1_data parameter; C1_data parameter; R2_data parameter; C2_data parameter; SoC_bp_ocv parameter; SoC_bp_ecm parameter; T_bp parameter; Q_nom_Ah parameter; dt parameter; ekf_params parameter; N_series input; SoC_pack output
function SoC_pack = ekf_soc_pack(V_pack, I_pack, T_pack, ...
    OCV_data, R0_data, R1_data, C1_data, R2_data, C2_data, ...
    SoC_bp_ocv, SoC_bp_ecm, T_bp, Q_nom_Ah, dt, ekf_params, N_series)
%EKF_SOC_PACK  Pack-level EKF for SoC estimation.
%
%   State vector: x = [SoC; V_RC1; V_RC2]
%   Measurement:  V_pack = N_series * (OCV(SoC,T) - I*R0 - V_RC1 - V_RC2)

    persistent x_hat P_mat initialized
    if isempty(initialized)
        x_hat = [ekf_params.SoC0; 0; 0];
        P_mat = diag([ekf_params.P0_SoC, 1e-4, 1e-4]);
        initialized = true;
    end

    Q_cov = diag([ekf_params.Q_SoC, ekf_params.Q_VRC1, ekf_params.Q_VRC2]);
    R_cov = ekf_params.R_V;

    SoC_k = x_hat(1);
    VRC1  = x_hat(2);
    VRC2  = x_hat(3);

    % --- Lookup ECM parameters at (SoC_k, T_pack) ---
    R0 = interp2_lut(SoC_bp_ecm, T_bp, R0_data, SoC_k * 100, T_pack);
    R1 = interp2_lut(SoC_bp_ecm, T_bp, R1_data, SoC_k * 100, T_pack);
    C1 = interp2_lut(SoC_bp_ecm, T_bp, C1_data, SoC_k * 100, T_pack);
    R2 = interp2_lut(SoC_bp_ecm, T_bp, R2_data, SoC_k * 100, T_pack);
    C2 = interp2_lut(SoC_bp_ecm, T_bp, C2_data, SoC_k * 100, T_pack);

    a1 = exp(-dt / (R1 * C1));
    a2 = exp(-dt / (R2 * C2));

    % --- Predict -------------------------------------------------------
    SoC_pred = SoC_k - (I_pack * dt) / (Q_nom_Ah * 3600);
    VRC1_pred = a1 * VRC1 + R1 * (1 - a1) * I_pack;
    VRC2_pred = a2 * VRC2 + R2 * (1 - a2) * I_pack;

    F      = [1, 0, 0;  0, a1, 0;  0, 0, a2];
    P_pred = F * P_mat * F' + Q_cov;

    % --- Update --------------------------------------------------------
    OCV_pred = interp2_lut(SoC_bp_ocv, T_bp, OCV_data, SoC_pred * 100, T_pack);
    V_pred   = N_series * (OCV_pred - I_pack * R0 - VRC1_pred - VRC2_pred);

    dOCV = numerical_dOCV(SoC_bp_ocv, T_bp, OCV_data, SoC_pred * 100, T_pack);
    H    = [N_series * dOCV * 100, -N_series, -N_series];

    S = H * P_pred * H' + R_cov;
    K = P_pred * H' / S;

    x_hat = [SoC_pred; VRC1_pred; VRC2_pred] + K * (V_pack - V_pred);
    P_mat = (eye(3) - K * H) * P_pred;

    SoC_pack = max(0, min(1, x_hat(1)));
end

function v = interp2_lut(xbp, ybp, data, xq, yq)
%INTERP2_LUT  Codegen-safe bilinear interpolation on a 2-D LUT.
    xq = max(xbp(1), min(xbp(end), xq));
    yq = max(ybp(1), min(ybp(end), yq));
    ix = int32(1);
    for k = 1:int32(numel(xbp) - 1)
        if xq >= xbp(k), ix = k; end
    end
    iy = int32(1);
    for k = 1:int32(numel(ybp) - 1)
        if yq >= ybp(k), iy = k; end
    end
    ix2 = min(ix + 1, int32(numel(xbp)));
    iy2 = min(iy + 1, int32(numel(ybp)));
    fx = 0; if ix ~= ix2, fx = (xq - xbp(ix)) / (xbp(ix2) - xbp(ix)); end
    fy = 0; if iy ~= iy2, fy = (yq - ybp(iy)) / (ybp(iy2) - ybp(iy)); end
    v = data(ix, iy)  * (1-fx) * (1-fy) + data(ix2, iy)  * fx * (1-fy) + ...
        data(ix, iy2) * (1-fx) *    fy  + data(ix2, iy2) * fx *    fy;
end

% -------------------------------------------------------------------------

function dv = numerical_dOCV(xbp, ybp, data, xq, yq)
%NUMERICAL_DOCV  Central-difference dOCV/dSoC [V/%].
    ds = 0.5;
    dv = (interp2_lut(xbp, ybp, data, xq + ds, yq) - ...
          interp2_lut(xbp, ybp, data, xq - ds, yq)) / (2 * ds);
end

== matlab function bms_master/Signal_Aggregator/Decode_Fault_Flags/decode_bits ==
  data: flags_8 input; OV_sev output; UV_sev output; OT_sev output; UT_sev output
function [OV_sev, UV_sev, OT_sev, UT_sev] = decode_bits(flags_8)
%#codegen
  ff = uint8(flags_8);
  OV_sev = double(bitand(ff, uint8(3)));
  UV_sev = double(bitand(bitshift(ff, -2), uint8(3)));
  OT_sev = double(bitand(bitshift(ff, -4), uint8(3)));
  UT_sev = double(bitand(bitshift(ff, -6), uint8(3)));
end

== stateflow chart bms_master/Fault_Severity_FSM ==
  settings: updateMethod=DISCRETE  sampleTime=0.1
  state Idle
    en : fault_severity = 0; shutdown_cmd = 0;
  state Warning
    en : fault_severity = 1; shutdown_cmd = 0;
  state Shutdown
    en : fault_severity = 3; shutdown_cmd = 1;
  state Derating
    en : fault_severity = 2; shutdown_cmd = 0;
  (default) -> Idle
  Idle -> Warning [order 1] : [max([max_V_sev, max_T_sev, I_sev, watchdog_sev]) >= 1]
  Warning -> Idle [order 2] : [max([max_V_sev, max_T_sev, I_sev, watchdog_sev]) == 0]
  Idle -> Shutdown [order 2] : [hw_fault]
  Warning -> Shutdown [order 3] : [max([max_V_sev, max_T_sev, I_sev, watchdog_sev]) >= 3 || hw_fault]
  Derating -> Warning [order 2] : [max([max_V_sev, max_T_sev, I_sev, watchdog_sev]) <= 1 && ~hw_fault]
  Warning -> Derating [order 1] : [max( [max_V_sev, max_T_sev, I_sev, watchdog_sev]) >= 2]
  Derating -> Shutdown [order 1] : [max([max_V_sev, max_T_sev, I_sev, watchdog_sev]) >= 3 || hw_fault]
  data: max_V_sev input double; max_T_sev input double; I_sev input double; hw_fault input boolean; watchdog_sev input double; fault_severity output double; shutdown_cmd output double
